simulink model "sim_control_discrete_distance_angle"  (R2017a)
settings: Solver=VariableStepAuto  StartTime=0.0  StopTime=200  RelTol=1e-3
values from neighbouring files (symbols this model uses):
  Coeffdd = cell2mat(den)    [control_speed.m]    (also in motor_model.m)
  CoeffKdd = cell2mat(den)    [motor_model.m]
  CoeffKdn = cell2mat(num)    [motor_model.m]
  Coeffnd = cell2mat(num)    [control_speed.m]    (also in motor_model.m)
  Tech = 1/fech    (= 0.00516525128054)    [control_speed.m]    (also in motor_model.m)
settings Model: Creator=hugo  LastModifiedBy=hugo

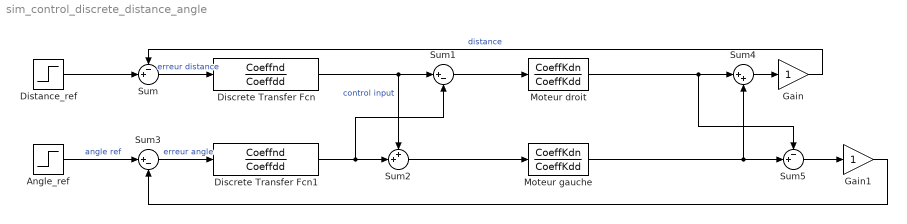
== system sim_control_discrete_distance_angle ==
  Angle_ref : Step  Time=2  After=600  SampleTime=0
  Discrete Transfer Fcn : DiscreteTransferFcn  Numerator=Coeffnd  Denominator=Coeffdd  SampleTime=Tech
  Discrete Transfer Fcn1 : DiscreteTransferFcn  Numerator=Coeffnd  Denominator=Coeffdd  SampleTime=Tech
  Distance_ref : Step  Time=6  After=5027  SampleTime=0
  Gain : Gain
  Gain1 : Gain
  Moteur droit : DiscreteTransferFcn  Numerator=CoeffKdn  Denominator=CoeffKdd  SampleTime=Tech
  Moteur gauche : DiscreteTransferFcn  Numerator=CoeffKdn  Denominator=CoeffKdd  SampleTime=Tech
  Sum : Sum  Inputs=-+|
  Sum1 : Sum  Inputs=|+-
  Sum2 : Sum  Inputs=++|
  Sum3 : Sum  Inputs=|+-
  Sum4 : Sum  Inputs=|++
  Sum5 : Sum  Inputs=-+|
  wires:
  Moteur droit/1 -> Sum5/1, Sum4/1
  Sum3/1 -> Discrete Transfer Fcn1/1  "erreur angle"
  Sum/1 -> Discrete Transfer Fcn/1  "erreur distance"
  Angle_ref/1 -> Sum3/1  "angle ref"
  Gain1/1 -> Sum3/2
  Sum2/1 -> Moteur gauche/1
  Sum1/1 -> Moteur droit/1
  Distance_ref/1 -> Sum/2
  Discrete Transfer Fcn/1 -> Sum2/1, Sum1/1  "control input"
  Discrete Transfer Fcn1/1 -> Sum1/2, Sum2/2
  Gain/1 -> Sum/1  "distance"
  Moteur gauche/1 -> Sum5/2, Sum4/2
  Sum4/1 -> Gain/1
  Sum5/1 -> Gain1/1
